simulink model "power_window"  (R2020b)
settings: Solver=VariableStepAuto  StartTime=0.0  StopTime=10.0  RelTol=1e-3
settings Model: Creator=Varun  LastModifiedBy=Varun

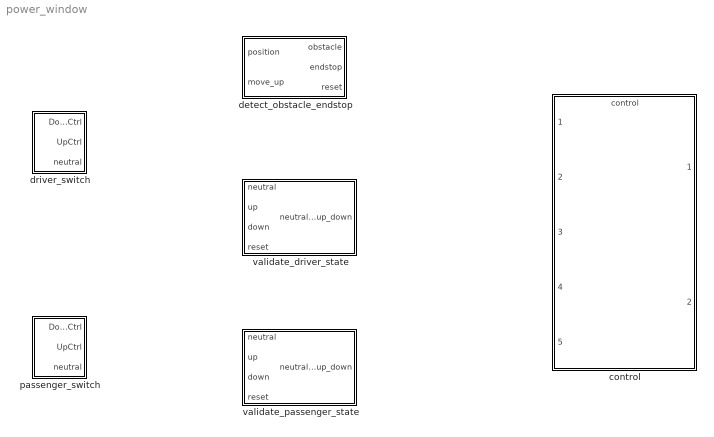
== system power_window ==
  control : ModelReference  ModelNameDialog=control  SimulationMode=Normal  ModelReferenceVersion=1.11
  detect_obstacle_endstop : Subsystem
  driver_switch : Subsystem
  passenger_switch : Subsystem
  validate_driver_state : Subsystem
  validate_passenger_state : Subsystem

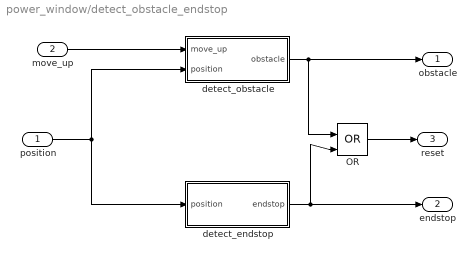
== system power_window/detect_obstacle_endstop ==
  position : Inport
  move_up : Inport  Port=2
  OR : Logic  Operator=OR  IconShape=distinctive  AllPortsSameDT=off  OutDataTypeStr=boolean
  detect_endstop : Subsystem
  detect_obstacle : Subsystem
  obstacle : Outport
  endstop : Outport  Port=2
  reset : Outport  Port=3
  wires:
  position/1 -> detect_obstacle/2(position), detect_endstop/1(position)
  move_up/1 -> detect_obstacle/1(move_up)
  detect_obstacle/1(obstacle) -> OR/1, obstacle/1
  detect_endstop/1(endstop) -> OR/2, endstop/1
  OR/1 -> reset/1

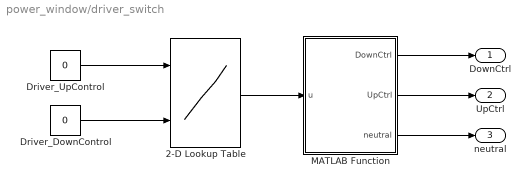
== system power_window/driver_switch ==
  2-D Lookup Table : Lookup_n-D  BreakpointsForDimension1=[0:1]  BreakpointsForDimension2=[0:1]  Table=[0 -1;1 0]  InternalRulePriority=Speed  RndMeth=Simplest  InputSameDT=on
      settings: InputPortMap=u0,u1
  Driver_DownControl : Constant  Value=0
  Driver_UpControl : Constant  Value=0
  MATLAB Function : MATLAB Function  TreatAsAtomicUnit=on
  DownCtrl : Outport
  UpCtrl : Outport  Port=2
  neutral : Outport  Port=3
  wires:
  MATLAB Function/1(DownCtrl) -> DownCtrl/1
  Driver_DownControl/1 -> 2-D Lookup Table/2
  MATLAB Function/2(UpCtrl) -> UpCtrl/1
  MATLAB Function/3(neutral) -> neutral/1
  Driver_UpControl/1 -> 2-D Lookup Table/1
  2-D Lookup Table/1 -> MATLAB Function/1(u)

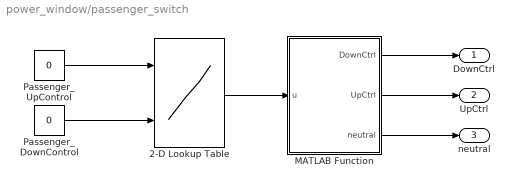
== system power_window/passenger_switch ==
  2-D Lookup Table : Lookup_n-D  BreakpointsForDimension1=[0:1]  BreakpointsForDimension2=[0:1]  Table=[0 -1;1 0]  InternalRulePriority=Speed  RndMeth=Simplest  InputSameDT=on
      settings: InputPortMap=u0,u1
  MATLAB Function : MATLAB Function  TreatAsAtomicUnit=on
  Passenger_DownControl : Constant  Value=0
  Passenger_UpControl : Constant  Value=0
  DownCtrl : Outport
  UpCtrl : Outport  Port=2
  neutral : Outport  Port=3
  wires:
  2-D Lookup Table/1 -> MATLAB Function/1(u)
  Passenger_UpControl/1 -> 2-D Lookup Table/1
  MATLAB Function/3(neutral) -> neutral/1
  MATLAB Function/2(UpCtrl) -> UpCtrl/1
  Passenger_DownControl/1 -> 2-D Lookup Table/2
  MATLAB Function/1(DownCtrl) -> DownCtrl/1

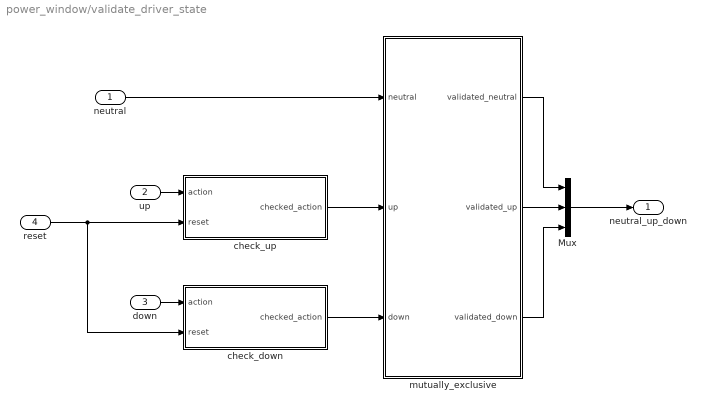
== system power_window/validate_driver_state ==
  neutral : Inport
  up : Inport  Port=2
  down : Inport  Port=3
  reset : Inport  Port=4
  Mux : Mux  Inputs=3
  check_down : Subsystem
  check_up : Subsystem
  mutually_exclusive : Subsystem
  neutral_up_down : Outport
  wires:
  up/1 -> check_up/1(action)
  reset/1 -> check_down/2(reset), check_up/2(reset)
  down/1 -> check_down/1(action)
  check_down/1(checked_action) -> mutually_exclusive/3(down)
  check_up/1(checked_action) -> mutually_exclusive/2(up)
  neutral/1 -> mutually_exclusive/1(neutral)
  Mux/1 -> neutral_up_down/1
  mutually_exclusive/1(validated_neutral) -> Mux/1
  mutually_exclusive/3(validated_down) -> Mux/3
  mutually_exclusive/2(validated_up) -> Mux/2

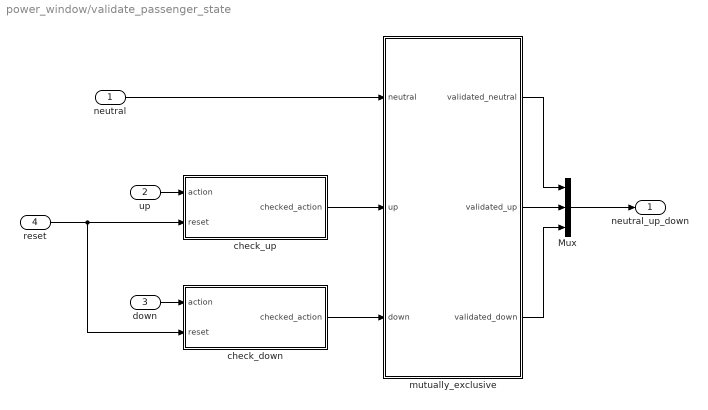
== system power_window/validate_passenger_state ==
  neutral : Inport
  up : Inport  Port=2
  down : Inport  Port=3
  reset : Inport  Port=4
  Mux : Mux  Inputs=3
  check_down : Subsystem
  check_up : Subsystem
  mutually_exclusive : Subsystem
  neutral_up_down : Outport
  wires:
  up/1 -> check_up/1(action)
  reset/1 -> check_down/2(reset), check_up/2(reset)
  down/1 -> check_down/1(action)
  check_down/1(checked_action) -> mutually_exclusive/3(down)
  check_up/1(checked_action) -> mutually_exclusive/2(up)
  neutral/1 -> mutually_exclusive/1(neutral)
  Mux/1 -> neutral_up_down/1
  mutually_exclusive/1(validated_neutral) -> Mux/1
  mutually_exclusive/3(validated_down) -> Mux/3
  mutually_exclusive/2(validated_up) -> Mux/2

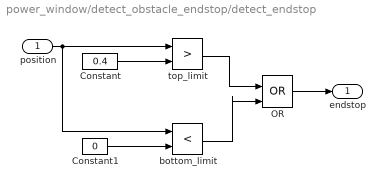
== system power_window/detect_obstacle_endstop/detect_endstop ==
  position : Inport
  Constant : Constant  Value=0.4
  Constant1 : Constant  Value=0
  OR : Logic  Operator=OR  IconShape=distinctive  AllPortsSameDT=off  OutDataTypeStr=boolean
  bottom_limit : RelationalOperator  Operator=<  OutDataTypeStr=boolean  RndMeth=Simplest
  top_limit : RelationalOperator  Operator=>  OutDataTypeStr=boolean  RndMeth=Simplest
  endstop : Outport
  wires:
  position/1 -> bottom_limit/1, top_limit/1
  Constant/1 -> top_limit/2
  OR/1 -> endstop/1
  top_limit/1 -> OR/1
  bottom_limit/1 -> OR/2
  Constant1/1 -> bottom_limit/2

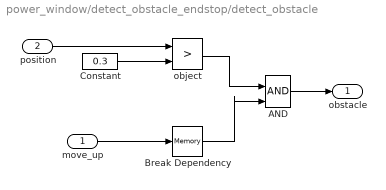
== system power_window/detect_obstacle_endstop/detect_obstacle ==
  move_up : Inport
  position : Inport  Port=2
  AND : Logic  IconShape=distinctive  AllPortsSameDT=off  OutDataTypeStr=boolean
  Break Dependency : Memory
  Constant : Constant  Value=0.3
  object : RelationalOperator  Operator=>  OutDataTypeStr=boolean  RndMeth=Simplest
  obstacle : Outport
  wires:
  object/1 -> AND/1
  AND/1 -> obstacle/1
  Constant/1 -> object/2
  position/1 -> object/1
  move_up/1 -> Break Dependency/1
  Break Dependency/1 -> AND/2

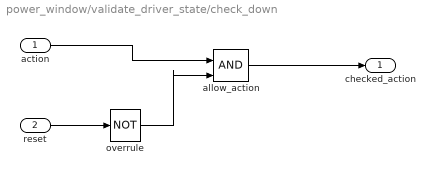
== system power_window/validate_driver_state/check_down ==
  action : Inport
  reset : Inport  Port=2
  allow_action : Logic  IconShape=distinctive  AllPortsSameDT=off  OutDataTypeStr=boolean
  overrule : Logic  Operator=NOT  IconShape=distinctive  AllPortsSameDT=off  OutDataTypeStr=boolean
  checked_action : Outport
  wires:
  action/1 -> allow_action/1
  overrule/1 -> allow_action/2
  allow_action/1 -> checked_action/1
  reset/1 -> overrule/1

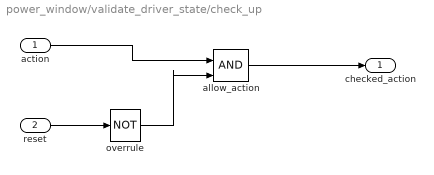
== system power_window/validate_driver_state/check_up ==
  action : Inport
  reset : Inport  Port=2
  allow_action : Logic  IconShape=distinctive  AllPortsSameDT=off  OutDataTypeStr=boolean
  overrule : Logic  Operator=NOT  IconShape=distinctive  AllPortsSameDT=off  OutDataTypeStr=boolean
  checked_action : Outport
  wires:
  reset/1 -> overrule/1
  allow_action/1 -> checked_action/1
  overrule/1 -> allow_action/2
  action/1 -> allow_action/1

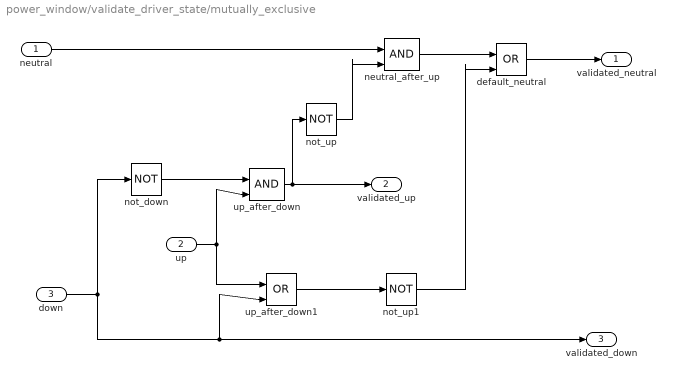
== system power_window/validate_driver_state/mutually_exclusive ==
  neutral : Inport
  up : Inport  Port=2
  down : Inport  Port=3
  default_neutral : Logic  Operator=OR  IconShape=distinctive  AllPortsSameDT=off  OutDataTypeStr=boolean
  neutral_after_up : Logic  IconShape=distinctive  AllPortsSameDT=off  OutDataTypeStr=boolean
  not_down : Logic  Operator=NOT  IconShape=distinctive  AllPortsSameDT=off  OutDataTypeStr=boolean
  not_up : Logic  Operator=NOT  IconShape=distinctive  AllPortsSameDT=off  OutDataTypeStr=boolean
  not_up1 : Logic  Operator=NOT  IconShape=distinctive  AllPortsSameDT=off  OutDataTypeStr=boolean
  up_after_down : Logic  IconShape=distinctive  AllPortsSameDT=off  OutDataTypeStr=boolean
  up_after_down1 : Logic  Operator=OR  IconShape=distinctive  AllPortsSameDT=off  OutDataTypeStr=boolean
  validated_neutral : Outport
  validated_up : Outport  Port=2
  validated_down : Outport  Port=3
  wires:
  neutral/1 -> neutral_after_up/1
  neutral_after_up/1 -> default_neutral/1
  default_neutral/1 -> validated_neutral/1
  not_up/1 -> neutral_after_up/2
  not_down/1 -> up_after_down/1
  up/1 -> up_after_down1/1, up_after_down/2
  down/1 -> validated_down/1, up_after_down1/2, not_down/1
  up_after_down1/1 -> not_up1/1
  not_up1/1 -> default_neutral/2
  up_after_down/1 -> not_up/1, validated_up/1

== system power_window/validate_passenger_state/check_down ==
  action : Inport
  reset : Inport  Port=2
  allow_action : Logic  IconShape=distinctive  AllPortsSameDT=off  OutDataTypeStr=boolean
  overrule : Logic  Operator=NOT  IconShape=distinctive  AllPortsSameDT=off  OutDataTypeStr=boolean
  checked_action : Outport
  wires:
  action/1 -> allow_action/1
  overrule/1 -> allow_action/2
  allow_action/1 -> checked_action/1
  reset/1 -> overrule/1

== system power_window/validate_passenger_state/check_up ==
  action : Inport
  reset : Inport  Port=2
  allow_action : Logic  IconShape=distinctive  AllPortsSameDT=off  OutDataTypeStr=boolean
  overrule : Logic  Operator=NOT  IconShape=distinctive  AllPortsSameDT=off  OutDataTypeStr=boolean
  checked_action : Outport
  wires:
  reset/1 -> overrule/1
  allow_action/1 -> checked_action/1
  overrule/1 -> allow_action/2
  action/1 -> allow_action/1

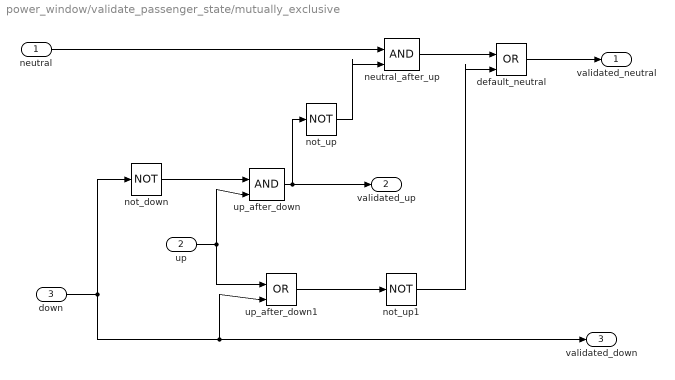
== system power_window/validate_passenger_state/mutually_exclusive ==
  neutral : Inport
  up : Inport  Port=2
  down : Inport  Port=3
  default_neutral : Logic  Operator=OR  IconShape=distinctive  AllPortsSameDT=off  OutDataTypeStr=boolean
  neutral_after_up : Logic  IconShape=distinctive  AllPortsSameDT=off  OutDataTypeStr=boolean
  not_down : Logic  Operator=NOT  IconShape=distinctive  AllPortsSameDT=off  OutDataTypeStr=boolean
  not_up : Logic  Operator=NOT  IconShape=distinctive  AllPortsSameDT=off  OutDataTypeStr=boolean
  not_up1 : Logic  Operator=NOT  IconShape=distinctive  AllPortsSameDT=off  OutDataTypeStr=boolean
  up_after_down : Logic  IconShape=distinctive  AllPortsSameDT=off  OutDataTypeStr=boolean
  up_after_down1 : Logic  Operator=OR  IconShape=distinctive  AllPortsSameDT=off  OutDataTypeStr=boolean
  validated_neutral : Outport
  validated_up : Outport  Port=2
  validated_down : Outport  Port=3
  wires:
  neutral/1 -> neutral_after_up/1
  neutral_after_up/1 -> default_neutral/1
  default_neutral/1 -> validated_neutral/1
  not_up/1 -> neutral_after_up/2
  not_down/1 -> up_after_down/1
  up/1 -> up_after_down1/1, up_after_down/2
  down/1 -> validated_down/1, up_after_down1/2, not_down/1
  up_after_down1/1 -> not_up1/1
  not_up1/1 -> default_neutral/2
  up_after_down/1 -> not_up/1, validated_up/1

== matlab function power_window/driver_switch/MATLAB Function ==
  data: u input; DownCtrl output; UpCtrl output; neutral output
function [DownCtrl,UpCtrl,neutral] = fcn(u)
DownCtrl=0;UpCtrl=0;neutral=0;
if(u == -1)
    DownCtrl = 1;
elseif(u==1)
    UpCtrl=1;
else
    neutral = 1;
end
end

== matlab function power_window/passenger_switch/MATLAB Function ==
  data: u input; DownCtrl output; UpCtrl output; neutral output
function [DownCtrl,UpCtrl,neutral] = fcn(u)
DownCtrl=0;UpCtrl=0;neutral=0;
if(u == -1)
    DownCtrl = 1;
elseif(u==1)
    UpCtrl=1;
else
    neutral = 1;
end
end
